simulink model "Final Version"  (R2018a)
settings: Solver=VariableStepAuto  StartTime=0.0  StopTime=20  RelTol=1e-3
libraries: simulink x1
settings Model: Creator=MAFAZ  LastModifiedBy=MAFAZ

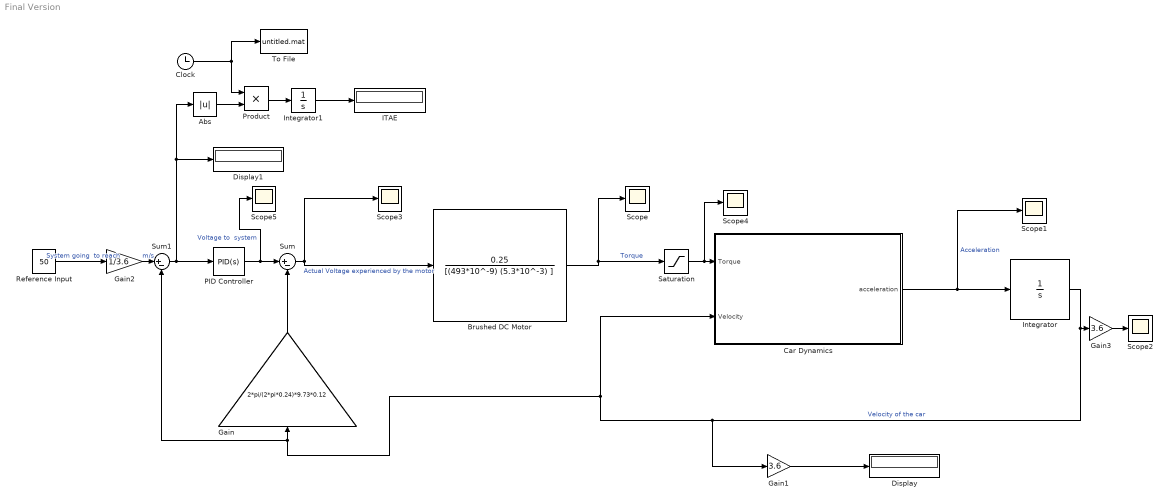
== system Final Version ==
  Abs : Abs
  Brushed DC Motor : TransferFcn  Numerator=[0.25]  Denominator=[(493*10^-9) (5.3*10^-3) ]
  Car Dynamics : MATLAB Function  TreatAsAtomicUnit=on
  Clock : Clock
  Display : Display
  Display1 : Display
  Gain : Gain  Gain=2*pi/(2*pi*0.24)*9.73*0.12
  Gain1 : Gain  Gain=3.6
  Gain2 : Gain  Gain=1/3.6
  Gain3 : Gain  Gain=3.6
  ITAE : Display
  Integrator : Integrator
  Integrator1 : Integrator
  PID Controller : simulink/Continuous/PID Controller  Controller=PID  TimeDomain=Continuous-time  SampleTime=-1  IntegratorMethod=Forward Euler  FilterMethod=Forward Euler  Form=Parallel  UseFilter=on  ControllerParametersSource=internal  P=1  I=10  D=0  N=100  InitialConditionSource=internal  InitialConditionForIntegrator=0  InitialConditionForFilter=0  ExternalReset=none  LimitOutput=on  UpperSaturationLimit=346  LowerSaturationLimit=0  LinearizeAsGain=on  AntiWindupMode=none  Kb=1  TrackingMode=off  Kt=1  PParamMin=[]  PParamMax=[]  IParamMin=[]  IParamMax=[]  DParamMin=[]  DParamMax=[]  NParamMin=[]  NParamMax=[]  KbParamMin=[]  KbParamMax=[]  KtParamMin=[]  KtParamMax=[]  POutMin=[]  POutMax=[]  IOutMin=[]  IOutMax=[]  DOutMin=[]  DOutMax=[]  NOutMin=[]  NOutMax=[]  KbOutMin=[]  KbOutMax=[]  KtOutMin=[]  KtOutMax=[]  IntegratorOutMin=[]  IntegratorOutMax=[]  FilterOutMin=[]  FilterOutMax=[]  SumOutMin=[]  SumOutMax=[]  SumI1OutMin=[]  SumI1OutMax=[]  SumI2OutMin=[]  SumI2OutMax=[]  SumI3OutMin=[]  SumI3OutMax=[]  SumDOutMin=[]  SumDOutMax=[]  SaturationOutMin=[]  SaturationOutMax=[]  IntegratorContinuousStateAttributes=''  IntegratorStateMustResolveToSignalObject=off  IntegratorRTWStateStorageClass=Auto  FilterContinuousStateAttributes=''  FilterStateMustResolveToSignalObject=off  FilterRTWStateStorageClass=Auto  DifferentiatorICPrevScaledInput=0  DifferentiatorOutMin=[]  DifferentiatorOutMax=[]  FilterDiffOutCoefMin=[]  FilterDiffOutCoefMax=[]  SumDenOutMin=[]  SumDenOutMax=[]  SumNumOutMin=[]  SumNumOutMax=[]  ReciprocalOutMin=[]  ReciprocalOutMax=[]  DivideOutMin=[]  DivideOutMax=[]  TunerSelectOption=Transfer Function Based (PID Tuner App)
  Product : Product
  Reference Input : Constant  Value=50
  Saturation : Saturate  UpperLimit=600  LowerLimit=0
  Scope{,1..5} (6 alike) : Scope
  Sum : Sum  Inputs=|+-
  Sum1 : Sum  Inputs=|+-
  To File : ToFile  SaveFormat=Timeseries
  wires:
  PID Controller/1 -> Scope5/1, Sum/1  "Voltage to  system"
  Gain/1 -> Sum/2
  Brushed DC Motor/1 -> Scope/1, Saturation/1  "Torque"
  Car Dynamics/1(acceleration) -> Scope1/1, Integrator/1  "Acceleration"
  Integrator/1 -> Gain3/1, Gain1/1, Sum1/2, Gain/1, Car Dynamics/2(Velocity)  "Velocity of the car"
  Sum/1 -> Scope3/1, Brushed DC Motor/1  "Actual Voltage experienced by the motor"
  Gain1/1 -> Display/1
  Saturation/1 -> Scope4/1, Car Dynamics/1(Torque)
  Reference Input/1 -> Gain2/1  "System going  to reach"
  Gain2/1 -> Sum1/1  "m/s"
  Sum1/1 -> Display1/1, Abs/1, PID Controller/1
  Gain3/1 -> Scope2/1
  Product/1 -> Integrator1/1
  Integrator1/1 -> ITAE/1
  Abs/1 -> Product/2
  Clock/1 -> To File/1, Product/1

== matlab function Final Version/Car Dynamics ==
  data: Torque input; acceleration output; Velocity input
function acceleration = fcn(Torque, Velocity)
acceleration = (40.5*Torque*0.6-413-0.3381*Velocity^2)/2108;
